simulink model "Test_GSM"  (R2018a)
settings: Solver=VariableStepAuto  StartTime=0.0  StopTime=Inf  RelTol=1e-3
settings Model: Creator=张紫薇  LastModifiedBy=lenovo

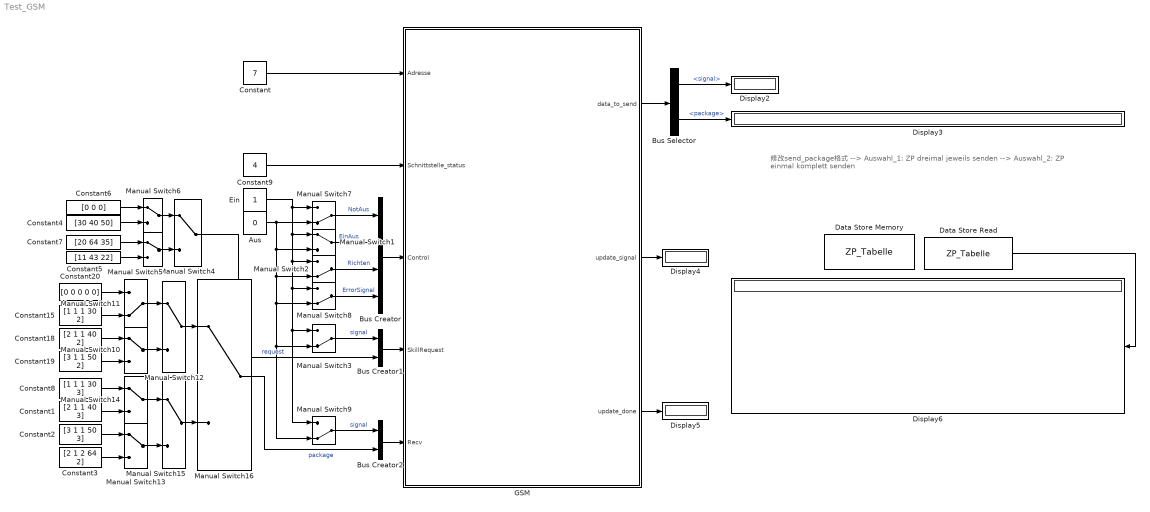
== system Test_GSM ==
  note: 修改send_package格式
      | --> Auswahl_1: ZP dreimal jeweils senden
      | --> Auswahl_2: ZP einmal komplett senden
  Aus : Constant  Value=0  OutDataTypeStr=boolean
  Bus Creator : BusCreator  Inputs=4
  Bus Creator1 : BusCreator  Inputs=2
  Bus Creator2 : BusCreator  Inputs=2
  Bus Selector : BusSelector  OutputSignals=signal,package
  Constant : Constant  Value=7  OutDataTypeStr=double
  Constant1 : Constant  Value=[2 1 1 40 3]
  Constant15 : Constant  Value=[1 1 1 30 2]
  Constant18 : Constant  Value=[2 1 1 40 2]
  Constant19 : Constant  Value=[3 1 1 50 2]
  Constant2 : Constant  Value=[3 1 1 50 3]
  Constant20 : Constant  Value=[0 0 0 0 0]
  Constant3 : Constant  Value=[2 1 2 64 2]
  Constant4 : Constant  Value=[30 40 50]
  Constant5 : Constant  Value=[11 43 22]
  Constant6 : Constant  Value=[0 0 0]
  Constant7 : Constant  Value=[20 64 35]
  Constant8 : Constant  Value=[1 1 1 30 3]
  Constant9 : Constant  Value=4  OutDataTypeStr=double
  Data Store Memory : DataStoreMemory  DataStoreName=ZP_Tabelle  ReadBeforeWriteMsg=warning  WriteAfterWriteMsg=warning  WriteAfterReadMsg=warning  InitialValue=zeros(10,7)  ShowAdditionalParam=off  OutDataTypeStr=double  Dimensions=[10 7]
  Data Store Read : DataStoreRead  DataStoreName=ZP_Tabelle
  Display{2..6} (5 alike) : Display
  Ein : Constant  OutDataTypeStr=boolean
  "GSM " : Subsystem
  Manual Switch{1,4..6,10,12..16} (10 alike) : ManualSwitch
  Manual Switch{2..3,7..9,11} (6 alike) : ManualSwitch  CurrentSetting=0
  wires:
  Bus Selector/1 -> Display2/1  "<signal>"
  Bus Selector/2 -> Display3/1  "<package>"
  Constant9/1 -> "GSM "/2(Schnittstelle_status)
  Constant20/1 -> Manual Switch11/1
  Constant15/1 -> Manual Switch11/2
  Constant18/1 -> Manual Switch10/1
  Constant19/1 -> Manual Switch10/2
  Manual Switch11/1 -> Manual Switch12/1
  Manual Switch10/1 -> Manual Switch12/2
  Data Store Read/1 -> Display6/1
  Constant5/1 -> Manual Switch5/2
  Constant7/1 -> Manual Switch5/1
  Constant4/1 -> Manual Switch6/2
  Manual Switch5/1 -> Manual Switch4/2
  Manual Switch6/1 -> Manual Switch4/1
  Constant6/1 -> Manual Switch6/1
  Aus/1 -> Manual Switch8/2, Manual Switch9/2, Manual Switch3/2, Manual Switch2/2, Manual Switch1/2, Manual Switch7/2
  Ein/1 -> Manual Switch8/1, Manual Switch9/1, Manual Switch3/1, Manual Switch2/1, Manual Switch1/1, Manual Switch7/1
  "GSM "/2(update_signal) -> Display4/1
  "GSM "/3(update_done) -> Display5/1
  Constant3/1 -> Manual Switch13/2
  Manual Switch13/1 -> Manual Switch15/2
  Constant8/1 -> Manual Switch14/1
  Constant1/1 -> Manual Switch14/2
  Manual Switch14/1 -> Manual Switch15/1
  Constant2/1 -> Manual Switch13/1
  Manual Switch12/1 -> Manual Switch16/1
  Manual Switch15/1 -> Manual Switch16/2
  Constant/1 -> "GSM "/1(Adresse)
  "GSM "/1(data_to_send) -> Bus Selector/1
  Manual Switch7/1 -> Bus Creator/1  "NotAus"
  Manual Switch1/1 -> Bus Creator/2  "EinAus"
  Manual Switch2/1 -> Bus Creator/3  "Richten"
  Manual Switch8/1 -> Bus Creator/4  "ErrorSignal"
  Bus Creator/1 -> "GSM "/3(Control)
  Manual Switch3/1 -> Bus Creator1/1  "signal"
  Manual Switch4/1 -> Bus Creator1/2  "request"
  Bus Creator1/1 -> "GSM "/4(SkillRequest)
  Manual Switch9/1 -> Bus Creator2/1  "signal"
  Manual Switch16/1 -> Bus Creator2/2  "package"
  Bus Creator2/1 -> "GSM "/5(Recv)

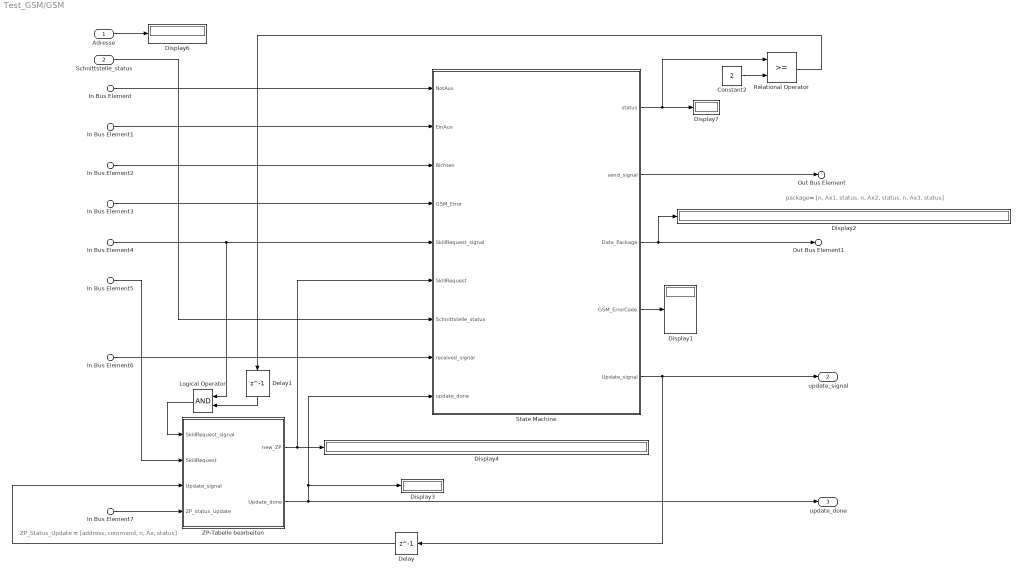
== system Test_GSM/GSM  ==
  note: package= [n, Ax1, status, n, Ax2, status, n, Ax3, status]
  note: ZP_Status_Update = [address, command, n, Ax, status]
  Adresse : Inport
  Schnittstelle_status : Inport  Port=2  OutDataTypeStr=double
  In Bus Element : Inport  Port=3  PortName=Control  Element=NotAus
  In Bus Element1 : Inport  Port=3  PortName=Control  Element=EinAus
  In Bus Element2 : Inport  Port=3  PortName=Control  Element=Richten
  In Bus Element3 : Inport  Port=3  PortName=Control  Element=ErrorSignal
  In Bus Element4 : Inport  Port=4  PortName=SkillRequest  Element=signal
  In Bus Element5 : Inport  Port=4  PortName=SkillRequest  Element=request
  In Bus Element6 : Inport  Port=5  PortName=Recv  Element=signal
  In Bus Element7 : Inport  Port=5  PortName=Recv  Element=package
  Constant2 : Constant  Value=2  OutDataTypeStr=double
  Delay : Delay  DelayLength=1
  Delay1 : Delay  DelayLength=1
  Display{1..4,6..7} (6 alike) : Display
  Logical Operator : Logic  AllPortsSameDT=off  OutDataTypeStr=boolean
  Relational Operator : RelationalOperator  OutDataTypeStr=boolean  RndMeth=Simplest
  State Machine : Stateflow chart  TreatAsAtomicUnit=on
  ZP-Tabelle bearbeiten : Subsystem
  Out Bus Element : Outport  PortName=data_to_send  Element=signal
  Out Bus Element1 : Outport  PortName=data_to_send  Element=package
  update_signal : Outport  Port=2  OutDataTypeStr=boolean
  update_done : Outport  Port=3
  wires:
  In Bus Element6/1 -> State Machine/8(received_signal)
  In Bus Element2/1 -> State Machine/3(Richten)
  State Machine/1(status) -> Relational Operator/1, Display7/1
  In Bus Element/1 -> State Machine/1(NotAus)
  In Bus Element1/1 -> State Machine/2(EinAus)
  Schnittstelle_status/1 -> State Machine/7(Schnittstelle_status)
  State Machine/4(GSM_ErrorCode) -> Display1/1
  In Bus Element4/1 -> Logical Operator/1, State Machine/5(SkillRequest_signal)
  In Bus Element5/1 -> ZP-Tabelle bearbeiten/2(SkillRequest)
  In Bus Element3/1 -> State Machine/4(GSM_Error)
  State Machine/2(send_signal) -> Out Bus Element/1
  State Machine/3(Data_Package) -> Out Bus Element1/1, Display2/1
  In Bus Element7/1 -> ZP-Tabelle bearbeiten/4(ZP_status_update)
  ZP-Tabelle bearbeiten/1(new_ZP) -> State Machine/6(SkillRequest), Display4/1
  ZP-Tabelle bearbeiten/2(Update_done) -> State Machine/9(update_done), Display3/1, update_done/1
  State Machine/5(Update_signal) -> update_signal/1, Delay/1
  Delay/1 -> ZP-Tabelle bearbeiten/3(Update_signal)
  Relational Operator/1 -> Delay1/1
  Logical Operator/1 -> ZP-Tabelle bearbeiten/1(SkillRequest_signal)
  Delay1/1 -> Logical Operator/2
  Constant2/1 -> Relational Operator/2
  Adresse/1 -> Display6/1

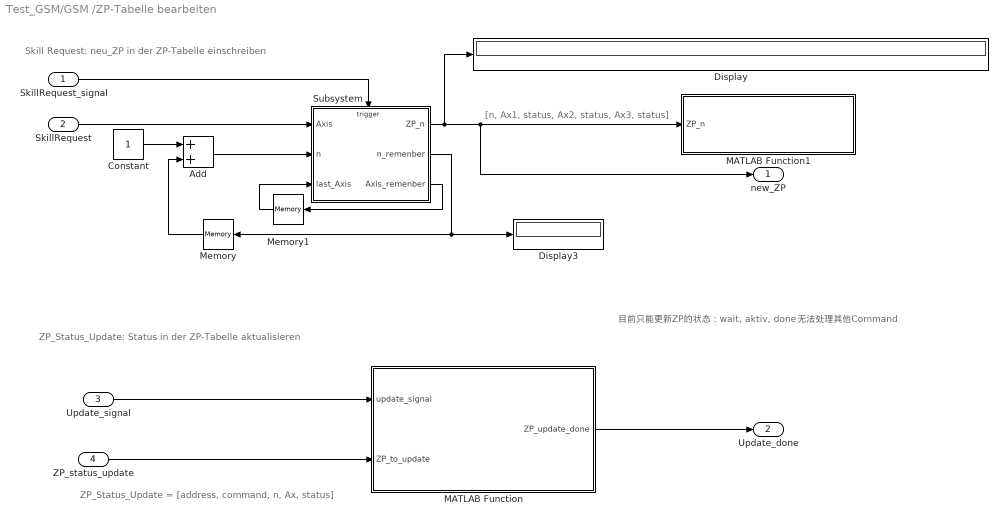
== system Test_GSM/GSM /ZP-Tabelle bearbeiten ==
  note: ZP_Status_Update = [address, command, n, Ax, status]
  note: Skill Request: neu_ZP in der ZP-Tabelle einschreiben
  note: ZP_Status_Update: Status in der ZP-Tabelle aktualisieren
  note: [n, Ax1, status, Ax2, status, Ax3, status]
  note: 目前只能更新ZP的状态：wait, aktiv, done
      | 无法处理其他Command
  SkillRequest_signal : Inport  OutDataTypeStr=boolean
  SkillRequest : Inport  Port=2  OutDataTypeStr=double  PortDimensions=3
  Update_signal : Inport  Port=3  OutDataTypeStr=boolean
  ZP_status_update : Inport  Port=4  OutDataTypeStr=double  PortDimensions=5
  Add : Sum
  Constant : Constant
  Display : Display
  Display3 : Display
  MATLAB Function : MATLAB Function  TreatAsAtomicUnit=on
  MATLAB Function1 : MATLAB Function  TreatAsAtomicUnit=on
  Memory : Memory
  Memory1 : Memory  InitialCondition=[0 0 0]
  Subsystem : Subsystem
  new_ZP : Outport
  Update_done : Outport  Port=2  OutDataTypeStr=boolean
  wires:
  Memory1/1 -> Subsystem/3(last_Axis)
  Subsystem/3(Axis_remenber) -> Memory1/1
  SkillRequest/1 -> Subsystem/1(Axis)
  Update_signal/1 -> MATLAB Function/1(update_signal)
  Add/1 -> Subsystem/2(n)
  ZP_status_update/1 -> MATLAB Function/2(ZP_to_update)
  MATLAB Function/1(ZP_update_done) -> Update_done/1
  Constant/1 -> Add/1
  SkillRequest_signal/1 -> Subsystem/Trigger
  Memory/1 -> Add/2
  Subsystem/2(n_remenber) -> Memory/1, Display3/1
  Subsystem/1(ZP_n) -> Display/1, MATLAB Function1/1(ZP_n), new_ZP/1

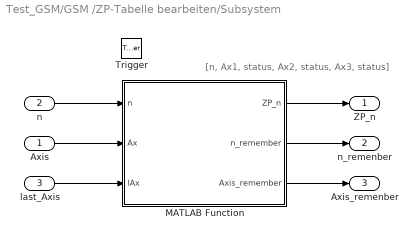
== system Test_GSM/GSM /ZP-Tabelle bearbeiten/Subsystem ==
  note: [n, Ax1, status, Ax2, status, Ax3, status]
  Axis : Inport
  n : Inport  Port=2
  last_Axis : Inport  Port=3
  Trigger : TriggerPort  VariantControl=Variant  PortDimensions=1
  MATLAB Function : MATLAB Function  TreatAsAtomicUnit=on
  ZP_n : Outport
  n_remenber : Outport  Port=2
  Axis_remenber : Outport  Port=3
  wires:
  n/1 -> MATLAB Function/1(n)
  Axis/1 -> MATLAB Function/2(Ax)
  MATLAB Function/1(ZP_n) -> ZP_n/1
  last_Axis/1 -> MATLAB Function/3(lAx)
  MATLAB Function/2(n_remember) -> n_remenber/1
  MATLAB Function/3(Axis_remember) -> Axis_remenber/1

== matlab function Test_GSM/GSM /ZP-Tabelle bearbeiten/Subsystem/MATLAB Function ==
  data: n input; ZP_n output double size=[1 7]; Ax input; lAx input; n_remember output; Axis_remember output
function [ZP_n, n_remember, Axis_remember] = Zielposition(n, Ax, lAx)

if ((Ax(1) == lAx(1)) && (Ax(2) == lAx(2)) && (Ax(3) == lAx(3))) == 0   %wiederholte Position filtern
    ZP_n = [n, Ax(1), 1, Ax(2), 1, Ax(3), 1];
    n_remember = n;
else
    ZP_n = [n-1, lAx(1), 1, lAx(2), 1, lAx(3),1];     %ZP_n ändert sich nicht
    n_remember = n-1;
end

Axis_remember = Ax;
end

== stateflow chart Test_GSM/GSM /State Machine ==
  settings: executeAtInitialization=1
  state Off
    entry: status = 0;
  state Error
    entry: status = -2;
  state Init
    entry: status = 1;
  state Run
    state Send_ZP
      entry:	status = 3;
      send_signal=SkillRequest_signal;
      Data_Package = SkillRequest;
    state Stand_By
      entry: status = 2;
    state ZP_Status_Update
      entry:	status = 4;
      Update_signal = received_signal;
    note: ZP_Status_Update = [address, command, n, Ax, status]
    note: received_package = [address, command, n, Ax, status]
    (default) -> Stand_By
    Stand_By -> Send_ZP [order 1] : [SkillRequest_signal]
    Send_ZP -> Stand_By : [~SkillRequest_signal]{send_signal=false;}
    ZP_Status_Update -> Stand_By : [update_done && ~received_signal]{Update_signal=false;}
    Stand_By -> ZP_Status_Update [order 2] : [received_signal && ~update_done]
  (default) -> Off
  Error -> Off [order 1] : [~EinAus]
  Off -> Error [order 2] : [EinAus && NotAus]
  Init -> Off [order 3] : [~EinAus]
  Off -> Init [order 1] : [EinAus && ~NotAus]
  Error -> Init [order 2] : [~GSM_Error && Richten] {GSM_ErrorCode=0;}
  Init -> Error [order 1] : [GSM_Error || NotAus]{GSM_ErrorCode=status}
  Run -> Init [order 2] : [Schnittstelle_status~=4 && ~GSM_Error]
  Init -> Run [order 2] : [Schnittstelle_status==4]
  Run -> Error [order 1] : [GSM_Error || NotAus]{GSM_ErrorCode=status}
  data: NotAus input boolean; EinAus input boolean; Richten input boolean; GSM_Error input boolean; SkillRequest_signal input boolean; SkillRequest input double size=7; Schnittstelle_status input double; status output double; send_signal output boolean; received_signal input boolean; update_done input boolean; Data_Package output double size=7; GSM_ErrorCode output double; Update_signal output boolean size=1

== matlab function Test_GSM/GSM /ZP-Tabelle bearbeiten/MATLAB Function ==
  data: update_signal input boolean; ZP_to_update input double size=5; ZP_update_done output boolean; ZP_Tabelle data_store_memory
%ZP_to_update = [address, command, n, Ax, status]

function ZP_update_done  = Status_Update(update_signal, ZP_to_update)

global ZP_Tabelle

N=0;
m=0;
n=0;

if update_signal == true
    address = ZP_to_update(1);
    m = 2 * address + 1;        % Matrix-Index berechnen
    n = ZP_to_update(3);        % ZP_n
    status = ZP_to_update(5);
    
    for i=1:10
        if ZP_Tabelle(i,1) == n
            N = i;              %ZP_N bestimmen
            break
        end
    end
    
    %N==1, status aktualisieren
    %N>1 && (status von ZP_N-1 == 'done'), status aktualisieren
    if (N == 1) || (N>1 && (ZP_Tabelle(N-1,3) == ZP_Tabelle(N-1,5) == ZP_Tabelle(N-1,7) == 3))
        ZP_Tabelle(N,m) = status;
        ZP_update_done = true;
    else        
        ZP_update_done = false;
    end
else
    ZP_update_done = false;
end

== matlab function Test_GSM/GSM /ZP-Tabelle bearbeiten/MATLAB Function1 ==
  data: ZP_n input; ZP_Tabelle data_store_memory
%ZP_n = [n, Ax1, status1, Ax2, status2, Ax3, status3];
%function ZP_newTable = new_ZP(ZP_n)

function new_ZP(ZP_n)

global ZP_Tabelle

m=0;
n = ZP_n(1);

for i = 1:10
    if ZP_Tabelle(i,1) == n
        break;
    end
    if ZP_Tabelle(i,1) == 0
        m=i;
        break
    end
end

if m ~= 0
    ZP_Tabelle(m,:) = ZP_n;
end

end
